simulink model "VTOL"  (R2015b)
settings: Solver=FixedStepAuto  StartTime=0.0  StopTime=30  FixedStep=sampleTime  RelTol=1e-3
InitFcn:
  | sampleTime = 0.01;
  | Ktd = 0.0526/1000;
  | Kdd = 0.0526/1000;
  | Lb = [0.27 0.27 0.27 0.27];
  | LbAssimetrico  = [0.27 0.27 0.18 0.36];
  | LbTeste  = [0.27 0.27 0.18 0.36];
  | Ixx = 0.0754483;
  | Iyy = 0.13642;
  | Izz = 0.2043333;
  | 
  | IXYZ = [Ixx 0 0; 0 Iyy 0; 0 0 Izz];
  | 
  | areaLateral = [0.0114398 0 0; 0 0.09533687 0; 0 0 0.33];
  | 
  | areaAsa = 0.243;
  | areaProfundor = 0.051;
  | densidadeAr = 1.2;
  | cdArrastoParasita = 1.5;
  | clAviao = 0.825;
  | cdAviao = 0.0743;
  | g = 9.8;
  | massa = 3;
  | velCruzeiro = 15;
  | 
  | inicioTransicao = 5;
  | 
  | global kroll
  | global kpitch
  | global kyaw
  | 
  | global kx
  | global ky
  | global kz
undefined symbols (not defined in the file or in its folder): DiscIntNeverNeededParam, kpitch, kroll, kx, ky, kyaw, kz
libraries: simulink x6, aerolibwind2 x1
settings Model: Creator=Avell-G1711  LastModifiedBy=Avell-G1711

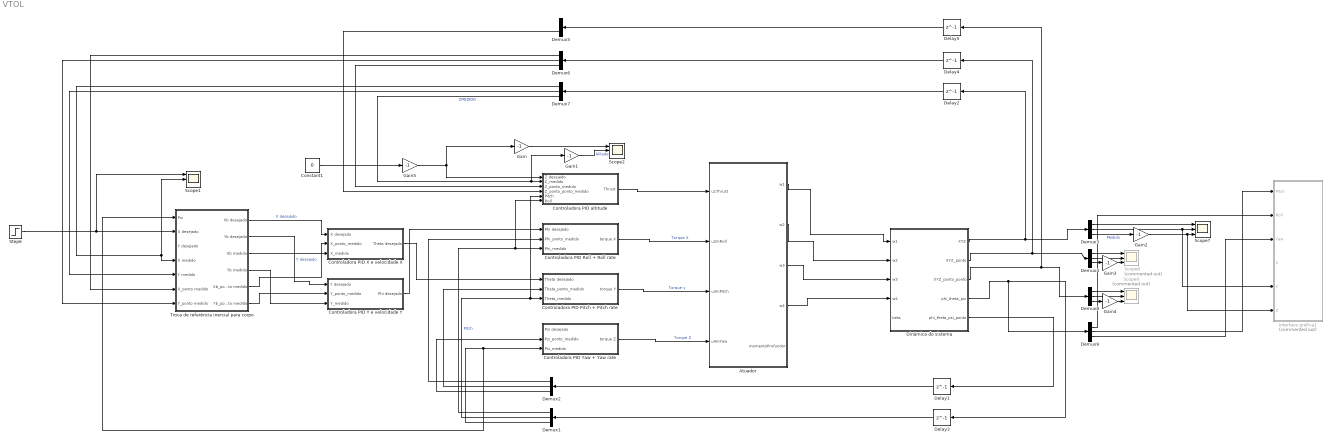
== system VTOL ==
  Atuador : Subsystem
  Constant1 : Constant  Value=0
  Controladora PID Pitch + Pitch rate : Subsystem
  Controladora PID Roll + Roll rate : Subsystem
  Controladora PID X e velocidade X : Subsystem
  Controladora PID Y e velocidade Y : Subsystem
  Controladora PID Yaw + Yaw rate : Subsystem
  Controladora PID altitude : Subsystem
  Delay{1..5} (5 alike) : Delay  DelayLength=1  InitialCondition=[0 0 0]
  Demux{1..9} (9 alike) : Demux  Outputs=3
  Dinâmica do sistema : Subsystem
  Gain{,1..5} (6 alike) : Gain  Gain=-1
  Interface gráfica1 : Subsystem  Commented=on  AncestorBlock=vampLib/Interface gráfica
  Scope1 : Scope  NumInputPorts=3
  Scope2 : Scope  NumInputPorts=3
  Scope7 : Scope  NumInputPorts=3
  Scope8 : Scope  Commented=on  NumInputPorts=3
  Scope9 : Scope  Commented=on  NumInputPorts=3
  Step6 : Step  Time=0  After=20  SampleTime=0
  Troca de referência inercial para corpo : Subsystem
  wires:
  Demux3/1 -> Scope7/1
  Demux3/3 -> Gain2/1  "Medido"
  Demux4/1 -> Scope8/1
  Demux4/2 -> Scope8/2
  Demux4/3 -> Gain3/1
  Dinâmica do sistema/2(XYZ_ponto) -> Delay4/1, Demux4/1
  Dinâmica do sistema/4(phi_theta_psi) -> Demux9/1, Delay3/1
  Dinâmica do sistema/5(phi_theta_psi_ponto) -> Delay1/1
  Delay1/1 -> Demux2/1
  Demux2/1 -> Controladora PID Roll + Roll rate/2(Phi_ponto_medido)
  Demux2/2 -> Controladora PID Pitch + Pitch rate/2(Theta_ponto_medido)
  Demux2/3 -> Controladora PID Yaw + Yaw rate/2(Psi_ponto_medido)
  Demux1/1 -> Controladora PID altitude/6(Roll), Controladora PID Roll + Roll rate/3(Phi_medido)
  Demux1/2 -> Controladora PID altitude/5(Pitch), Controladora PID Pitch + Pitch rate/3(Theta_medido)  "Pitch"
  Atuador/3(w3) -> Dinâmica do sistema/3(w3)
  Atuador/1(w1) -> Dinâmica do sistema/1(w1)
  Atuador/2(w2) -> Dinâmica do sistema/2(w2)
  Atuador/4(w4) -> Dinâmica do sistema/4(w4)
  Controladora PID Roll + Roll rate/1(torque X) -> Atuador/2(u2mRoll)  "Torque X"
  Controladora PID Pitch + Pitch rate/1(torque Y) -> Atuador/3(u3mPitch)  "Torque y"
  Controladora PID Yaw + Yaw rate/1(torque Z) -> Atuador/4(u4mYaw)  "Torque Z"
  Demux7/3 -> Controladora PID altitude/2(Z_medido), Gain1/1  "ZMEDIDO"
  Dinâmica do sistema/1(XYZ) -> Delay2/1, Demux3/1
  Delay5/1 -> Demux5/1
  Delay4/1 -> Demux6/1
  Delay2/1 -> Demux7/1
  Demux5/3 -> Controladora PID altitude/4(Z_ponto_ponto_medido)
  Demux6/3 -> Controladora PID altitude/3(Z_ponto_medido)
  Troca de referência inercial para corpo/1(Xb desejado) -> Controladora PID X e velocidade X/1(X desejado)  "X desejado"
  Troca de referência inercial para corpo/2(Yb desejado) -> Controladora PID Y e velocidade Y/1(Y desejado)  "Y desejado"
  Demux7/1 -> Troca de referência inercial para corpo/4(X medido), Scope1/2
  Demux6/1 -> Troca de referência inercial para corpo/6(X_ponto medido)
  Demux6/2 -> Troca de referência inercial para corpo/7(Y_ponto medido)
  Demux8/1 -> Scope9/1
  Demux8/2 -> Scope9/2
  Demux8/3 -> Gain4/1
  Dinâmica do sistema/3(XYZ_ponto_ponto) -> Demux8/1, Delay5/1
  Gain/1 -> Scope2/1
  Gain1/1 -> Scope2/2  "Alitude"
  Gain2/1 -> Interface gráfica1/6(Z), Scope7/3
  Gain3/1 -> Scope8/3
  Gain4/1 -> Scope9/3
  Troca de referência inercial para corpo/3(Xb medido) -> Controladora PID X e velocidade X/3(X_medido)
  Troca de referência inercial para corpo/4(Yb medido) -> Controladora PID Y e velocidade Y/3(Y_medido)
  Troca de referência inercial para corpo/5(Xb_ponto medido) -> Controladora PID X e velocidade X/2(X_ponto_medido)
  Troca de referência inercial para corpo/6(Yb_ponto medido) -> Controladora PID Y e velocidade Y/2(Y_ponto_medido)
  Demux9/1 -> Interface gráfica1/2(Roll)
  Demux9/3 -> Interface gráfica1/3(Yaw)
  Controladora PID altitude/1(Thrust) -> Atuador/1(u1Thrust)
  Delay3/1 -> Demux1/1
  Demux1/3 -> Troca de referência inercial para corpo/1(Psi), Controladora PID Yaw + Yaw rate/3(Psi_medido)
  Gain5/1 -> Controladora PID altitude/1(Z desejado), Gain/1
  Demux7/2 -> Troca de referência inercial para corpo/5(Y medido)
  Controladora PID X e velocidade X/1(Theta desejado) -> Controladora PID Pitch + Pitch rate/1(Theta desejado)
  Controladora PID Y e velocidade Y/1(Phi desejado) -> Controladora PID Roll + Roll rate/1(Phi desejado)
  Constant1/1 -> Gain5/1
  Demux3/2 -> Interface gráfica1/5(Y), Scope7/2
  Demux9/2 -> Interface gráfica1/1(Pitch)
  Step6/1 -> Troca de referência inercial para corpo/2(X desejado), Scope1/1

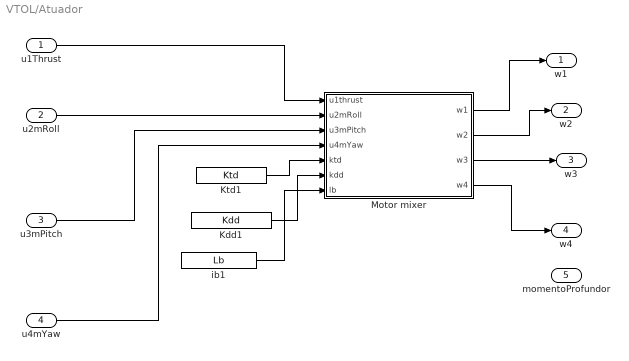
== system VTOL/Atuador ==
  u1Thrust : Inport
  u2mRoll : Inport  Port=2
  u3mPitch : Inport  Port=3
  u4mYaw : Inport  Port=4
  Kdd1 : Constant  Value=Kdd
  Ktd1 : Constant  Value=Ktd
  Motor mixer : MATLAB Function  TreatAsAtomicUnit=on
  ib1 : Constant  Value=Lb
  w1 : Outport
  w2 : Outport  Port=2
  w3 : Outport  Port=3
  w4 : Outport  Port=4
  momentoProfundor : Outport  Port=5
  wires:
  u3mPitch/1 -> Motor mixer/3(u3mPitch)
  ib1/1 -> Motor mixer/7(lb)
  Motor mixer/2(w2) -> w2/1
  Motor mixer/1(w1) -> w1/1
  u1Thrust/1 -> Motor mixer/1(u1thrust)
  Motor mixer/3(w3) -> w3/1
  Motor mixer/4(w4) -> w4/1
  u4mYaw/1 -> Motor mixer/4(u4mYaw)
  u2mRoll/1 -> Motor mixer/2(u2mRoll)
  Ktd1/1 -> Motor mixer/5(ktd)
  Kdd1/1 -> Motor mixer/6(kdd)
  ? -> momentoProfundor/1

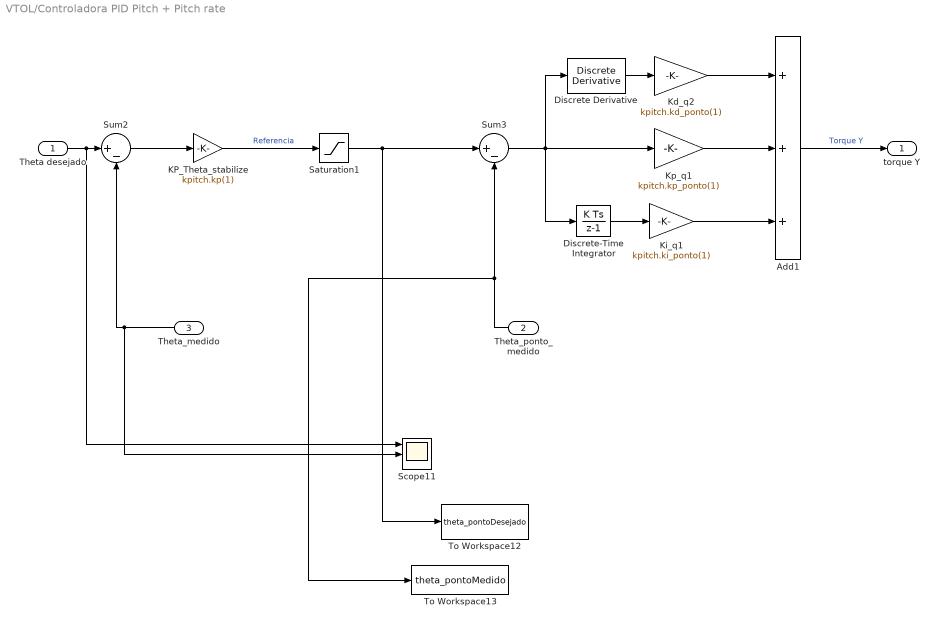
== system VTOL/Controladora PID Pitch + Pitch rate ==
  Theta desejado : Inport
  Theta_ponto_medido : Inport  Port=2
  Theta_medido : Inport  Port=3
  Add1 : Sum  Inputs=+++
  Discrete Derivative : simulink/Discrete/Discrete Derivative  gainval=1.0  ICPrevScaledInput=0.0  InputProcessing=Inherited  OutMin=[]  OutMax=[]  OutDataType=fixdt(1, 16)  OutScaling=2^-10  DoSatur=off
  Discrete-Time Integrator : DiscreteIntegrator  InitialConditionSetting=State (most efficient)  SampleTime=-1  ICPrevOutput=DiscIntNeverNeededParam  ICPrevScaledInput=DiscIntNeverNeededParam
  KP_Theta_stabilize : Gain  Gain=kpitch.kp(1)
  Kd_q2 : Gain  Gain=kpitch.kd_ponto(1)
  Ki_q1 : Gain  Gain=kpitch.ki_ponto(1)
  Kp_q1 : Gain  Gain=kpitch.kp_ponto(1)
  Saturation1 : Saturate  UpperLimit=2*pi  LowerLimit=-2*pi
  Scope11 : Scope  NumInputPorts=3
  Sum2 : Sum  Inputs=|+-
  Sum3 : Sum  Inputs=|+-
  To Workspace12 : ToWorkspace  VariableName=theta_pontoDesejado  SaveFormat=Timeseries  SampleTime=-1
  To Workspace13 : ToWorkspace  VariableName=theta_pontoMedido  SaveFormat=Timeseries  SampleTime=-1
  torque Y : Outport
  wires:
  Theta_ponto_medido/1 -> To Workspace13/1, Sum3/2
  Discrete-Time Integrator/1 -> Ki_q1/1
  Theta_medido/1 -> Scope11/2, Sum2/2
  Kd_q2/1 -> Add1/1
  Sum2/1 -> KP_Theta_stabilize/1
  Ki_q1/1 -> Add1/3
  Discrete Derivative/1 -> Kd_q2/1
  Sum3/1 -> Discrete Derivative/1, Discrete-Time Integrator/1, Kp_q1/1
  Kp_q1/1 -> Add1/2
  Theta desejado/1 -> Scope11/1, Sum2/1
  KP_Theta_stabilize/1 -> Saturation1/1  "Referencia"
  Add1/1 -> torque Y/1  "Torque Y"
  Saturation1/1 -> To Workspace12/1, Sum3/1

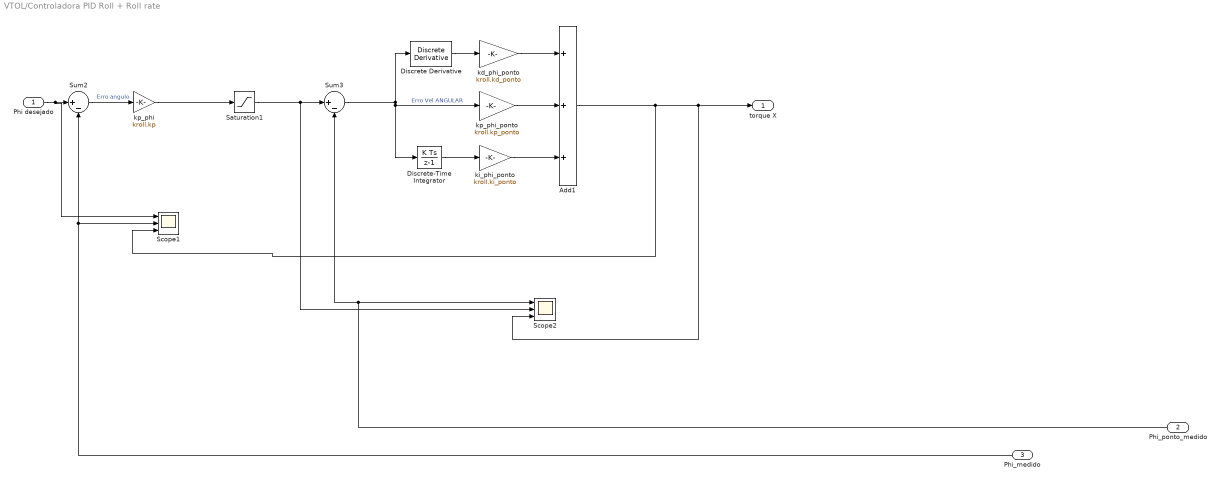
== system VTOL/Controladora PID Roll + Roll rate ==
  Phi desejado : Inport
  Phi_ponto_medido : Inport  Port=2
  Phi_medido : Inport  Port=3
  Add1 : Sum  Inputs=+++
  Discrete Derivative : simulink/Discrete/Discrete Derivative  gainval=1.0  ICPrevScaledInput=0.0  InputProcessing=Inherited  OutMin=[]  OutMax=[]  OutDataType=fixdt(1, 16)  OutScaling=2^-10  DoSatur=off
  Discrete-Time Integrator : DiscreteIntegrator  InitialConditionSetting=State (most efficient)  SampleTime=-1  ICPrevOutput=DiscIntNeverNeededParam  ICPrevScaledInput=DiscIntNeverNeededParam
  Saturation1 : Saturate  UpperLimit=2*pi  LowerLimit=-2*pi
  Scope1 : Scope  NumInputPorts=3
  Scope2 : Scope  NumInputPorts=3
  Sum2 : Sum  Inputs=|+-
  Sum3 : Sum  Inputs=|+-
  kd_phi_ponto : Gain  Gain=kroll.kd_ponto
  ki_phi_ponto : Gain  Gain=kroll.ki_ponto
  kp_phi : Gain  Gain=kroll.kp
  kp_phi_ponto : Gain  Gain=kroll.kp_ponto
  torque X : Outport
  wires:
  Phi_ponto_medido/1 -> Sum3/2, Scope2/1
  Discrete-Time Integrator/1 -> ki_phi_ponto/1
  Add1/1 -> Scope1/3, Scope2/3, torque X/1
  kd_phi_ponto/1 -> Add1/1
  Sum2/1 -> kp_phi/1  "Erro angulo"
  ki_phi_ponto/1 -> Add1/3
  Discrete Derivative/1 -> kd_phi_ponto/1
  kp_phi_ponto/1 -> Add1/2
  Phi desejado/1 -> Scope1/1, Sum2/1
  Sum3/1 -> Discrete-Time Integrator/1, kp_phi_ponto/1, Discrete Derivative/1  "Erro Vel ANGULAR"
  Phi_medido/1 -> Scope1/2, Sum2/2
  kp_phi/1 -> Saturation1/1
  Saturation1/1 -> Scope2/2, Sum3/1

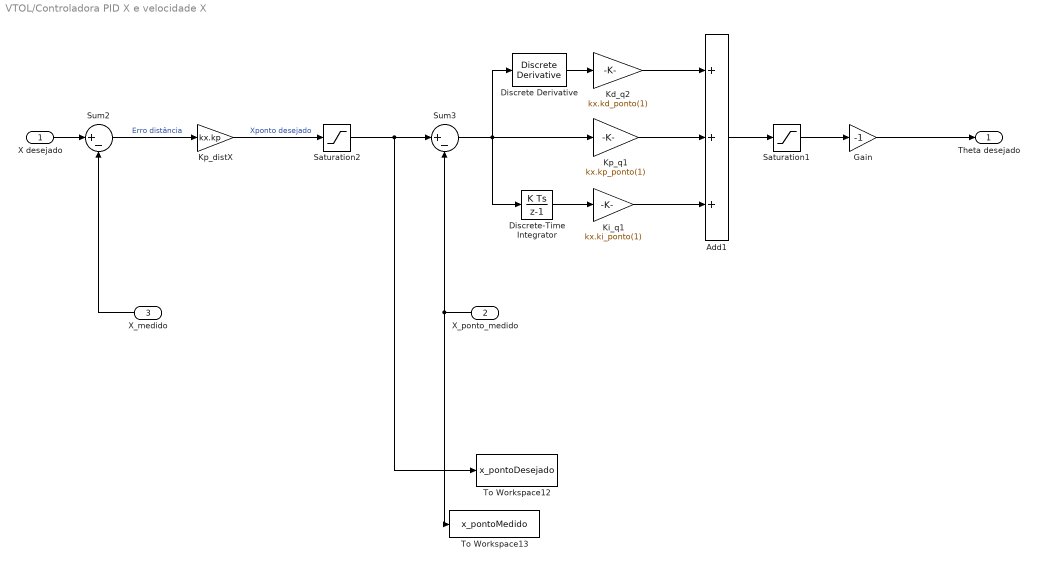
== system VTOL/Controladora PID X e velocidade X ==
  X desejado : Inport
  X_ponto_medido : Inport  Port=2
  X_medido : Inport  Port=3
  Add1 : Sum  Inputs=+++
  Discrete Derivative : simulink/Discrete/Discrete Derivative  gainval=1.0  ICPrevScaledInput=0.0  InputProcessing=Inherited  OutMin=[]  OutMax=[]  OutDataType=fixdt(1, 16)  OutScaling=2^-10  DoSatur=off
  Discrete-Time Integrator : DiscreteIntegrator  InitialConditionSetting=State (most efficient)  SampleTime=-1  ICPrevOutput=DiscIntNeverNeededParam  ICPrevScaledInput=DiscIntNeverNeededParam
  Gain : Gain  Gain=-1
  Kd_q2 : Gain  Gain=kx.kd_ponto(1)
  Ki_q1 : Gain  Gain=kx.ki_ponto(1)
  Kp_distX : Gain  Gain=kx.kp
  Kp_q1 : Gain  Gain=kx.kp_ponto(1)
  Saturation1 : Saturate  UpperLimit=0.7  LowerLimit=-0.7
  Saturation2 : Saturate  UpperLimit=4  LowerLimit=-4
  Sum2 : Sum  Inputs=|+-
  Sum3 : Sum  Inputs=|+-
  To Workspace12 : ToWorkspace  VariableName=x_pontoDesejado  SaveFormat=Timeseries  SampleTime=-1
  To Workspace13 : ToWorkspace  VariableName=x_pontoMedido  SaveFormat=Timeseries  SampleTime=-1
  Theta desejado : Outport
  wires:
  X_ponto_medido/1 -> Sum3/2, To Workspace13/1
  Discrete-Time Integrator/1 -> Ki_q1/1
  Add1/1 -> Saturation1/1
  Kd_q2/1 -> Add1/1
  Sum2/1 -> Kp_distX/1  "Erro distância"
  Ki_q1/1 -> Add1/3
  Discrete Derivative/1 -> Kd_q2/1
  Kp_q1/1 -> Add1/2
  X desejado/1 -> Sum2/1
  Kp_distX/1 -> Saturation2/1  "Xponto desejado"
  Sum3/1 -> Discrete Derivative/1, Discrete-Time Integrator/1, Kp_q1/1
  X_medido/1 -> Sum2/2
  Saturation1/1 -> Gain/1
  Saturation2/1 -> To Workspace12/1, Sum3/1
  Gain/1 -> Theta desejado/1

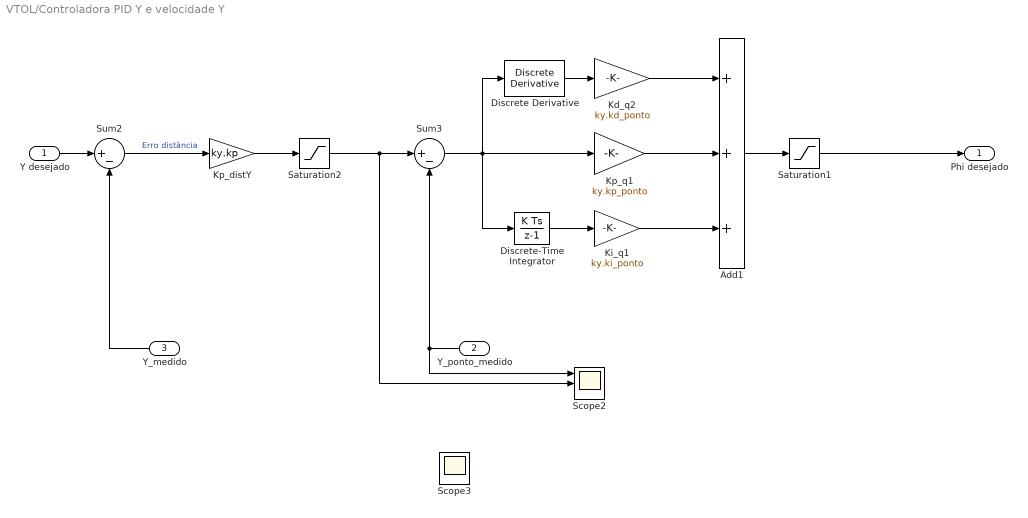
== system VTOL/Controladora PID Y e velocidade Y ==
  Y desejado : Inport
  Y_ponto_medido : Inport  Port=2
  Y_medido : Inport  Port=3
  Add1 : Sum  Inputs=+++
  Discrete Derivative : simulink/Discrete/Discrete Derivative  gainval=1.0  ICPrevScaledInput=0.0  InputProcessing=Inherited  OutMin=[]  OutMax=[]  OutDataType=fixdt(1, 16)  OutScaling=2^-10  DoSatur=off
  Discrete-Time Integrator : DiscreteIntegrator  InitialConditionSetting=State (most efficient)  SampleTime=-1  ICPrevOutput=DiscIntNeverNeededParam  ICPrevScaledInput=DiscIntNeverNeededParam
  Kd_q2 : Gain  Gain=ky.kd_ponto
  Ki_q1 : Gain  Gain=ky.ki_ponto
  Kp_distY : Gain  Gain=ky.kp
  Kp_q1 : Gain  Gain=ky.kp_ponto
  Saturation1 : Saturate  UpperLimit=0.7  LowerLimit=-0.7
  Saturation2 : Saturate  UpperLimit=4  LowerLimit=-4
  Scope2 : Scope  NumInputPorts=3
  Scope3 : Scope  NumInputPorts=3
  Sum2 : Sum  Inputs=|+-
  Sum3 : Sum  Inputs=|+-
  Phi desejado : Outport
  wires:
  Y_ponto_medido/1 -> Sum3/2, Scope2/1
  Discrete-Time Integrator/1 -> Ki_q1/1
  Add1/1 -> Saturation1/1
  Kd_q2/1 -> Add1/1
  Sum2/1 -> Kp_distY/1  "Erro distância"
  Ki_q1/1 -> Add1/3
  Discrete Derivative/1 -> Kd_q2/1
  Kp_q1/1 -> Add1/2
  Y desejado/1 -> Sum2/1
  Kp_distY/1 -> Saturation2/1
  Sum3/1 -> Discrete Derivative/1, Discrete-Time Integrator/1, Kp_q1/1
  Y_medido/1 -> Sum2/2
  Saturation2/1 -> Scope2/2, Sum3/1
  Saturation1/1 -> Phi desejado/1

== system VTOL/Controladora PID Yaw + Yaw rate ==
  Psi desejado : Inport
  Psi_ponto_medido : Inport  Port=2
  Psi_medido : Inport  Port=3
  Add1 : Sum  Inputs=+++
  Discrete Derivative : simulink/Discrete/Discrete Derivative  gainval=1.0  ICPrevScaledInput=0.0  InputProcessing=Inherited  OutMin=[]  OutMax=[]  OutDataType=fixdt(1, 16)  OutScaling=2^-10  DoSatur=off
  Discrete-Time Integrator : DiscreteIntegrator  InitialConditionSetting=State (most efficient)  SampleTime=-1  ICPrevOutput=DiscIntNeverNeededParam  ICPrevScaledInput=DiscIntNeverNeededParam
  KP_phi_stabilize1 : Gain  Gain=kyaw.kp
  Kd_q2 : Gain  Gain=kyaw.kd_ponto
  Ki_q1 : Gain  Gain=kyaw.ki_ponto
  Kp_q1 : Gain  Gain=kyaw.kp_ponto
  Sum2 : Sum  Inputs=|+-
  Sum3 : Sum  Inputs=|+-
  torque Z : Outport
  wires:
  Psi_ponto_medido/1 -> Sum3/2
  Discrete-Time Integrator/1 -> Ki_q1/1
  Psi_medido/1 -> Sum2/2
  Kd_q2/1 -> Add1/1
  Sum2/1 -> KP_phi_stabilize1/1
  Ki_q1/1 -> Add1/3
  Discrete Derivative/1 -> Kd_q2/1
  Sum3/1 -> Discrete Derivative/1, Discrete-Time Integrator/1, Kp_q1/1
  Kp_q1/1 -> Add1/2
  Psi desejado/1 -> Sum2/1
  KP_phi_stabilize1/1 -> Sum3/1  "Referencia"
  Add1/1 -> torque Z/1  "Torque Z"

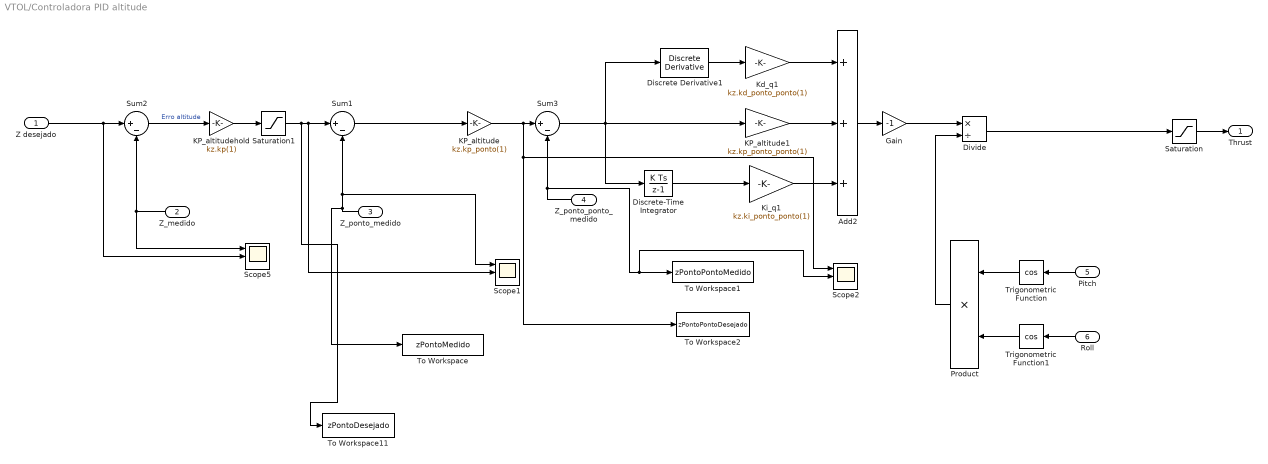
== system VTOL/Controladora PID altitude ==
  Z desejado : Inport
  Z_medido : Inport  Port=2
  Z_ponto_medido : Inport  Port=3
  Z_ponto_ponto_medido : Inport  Port=4
  Pitch : Inport  Port=5
  Roll : Inport  Port=6
  Add2 : Sum  Inputs=+++
  Discrete Derivative1 : simulink/Discrete/Discrete Derivative  gainval=1.0  ICPrevScaledInput=0.0  InputProcessing=Inherited  OutMin=[]  OutMax=[]  OutDataType=fixdt(1, 16)  OutScaling=2^-10  DoSatur=off
  Discrete-Time Integrator : DiscreteIntegrator  InitialConditionSetting=State (most efficient)  SampleTime=-1  ICPrevOutput=DiscIntNeverNeededParam  ICPrevScaledInput=DiscIntNeverNeededParam
  Divide : Product  Inputs=*/
  Gain : Gain  Gain=-1
  KP_altitude : Gain  Gain=kz.kp_ponto(1)
  KP_altitude1 : Gain  Gain=kz.kp_ponto_ponto(1)
  KP_altitudehold : Gain  Gain=kz.kp(1)
  Kd_q1 : Gain  Gain=kz.kd_ponto_ponto(1)
  Ki_q1 : Gain  Gain=kz.ki_ponto_ponto(1)
  Product : Product
  Saturation : Saturate  UpperLimit=53  LowerLimit=0
  Saturation1 : Saturate  UpperLimit=2  LowerLimit=-2
  Scope1 : Scope  NumInputPorts=3
  Scope2 : Scope  NumInputPorts=3
  Scope5 : Scope  NumInputPorts=3
  Sum1 : Sum  Inputs=|+-
  Sum2 : Sum  Inputs=|+-
  Sum3 : Sum  Inputs=|+-
  To Workspace : ToWorkspace  VariableName=zPontoMedido  SaveFormat=Timeseries  SampleTime=-1
  To Workspace1 : ToWorkspace  VariableName=zPontoPontoMedido  SaveFormat=Timeseries  SampleTime=-1
  To Workspace11 : ToWorkspace  VariableName=zPontoDesejado  SaveFormat=Timeseries  SampleTime=-1
  To Workspace2 : ToWorkspace  VariableName=zPontoPontoDesejado  SaveFormat=Timeseries  SampleTime=-1
  Trigonometric Function : Trigonometry  Operator=cos
  Trigonometric Function1 : Trigonometry  Operator=cos
  Thrust : Outport
  wires:
  Sum2/1 -> KP_altitudehold/1  "Erro altitude"
  Z desejado/1 -> Scope5/2, Sum2/1
  Z_medido/1 -> Sum2/2, Scope5/1
  Z_ponto_medido/1 -> To Workspace/1, Scope1/1, Sum1/2
  KP_altitudehold/1 -> Saturation1/1
  Sum1/1 -> KP_altitude/1
  KP_altitude/1 -> Scope2/1, To Workspace2/1, Sum3/1
  Z_ponto_ponto_medido/1 -> Scope2/2, To Workspace1/1, Sum3/2
  KP_altitude1/1 -> Add2/2
  Discrete Derivative1/1 -> Kd_q1/1
  Kd_q1/1 -> Add2/1
  Discrete-Time Integrator/1 -> Ki_q1/1
  Ki_q1/1 -> Add2/3
  Sum3/1 -> Discrete-Time Integrator/1, KP_altitude1/1, Discrete Derivative1/1
  Pitch/1 -> Trigonometric Function/1
  Roll/1 -> Trigonometric Function1/1
  Product/1 -> Divide/2
  Add2/1 -> Gain/1
  Trigonometric Function/1 -> Product/1
  Trigonometric Function1/1 -> Product/2
  Gain/1 -> Divide/1
  Saturation/1 -> Thrust/1
  Divide/1 -> Saturation/1
  Saturation1/1 -> To Workspace11/1, Scope1/2, Sum1/1

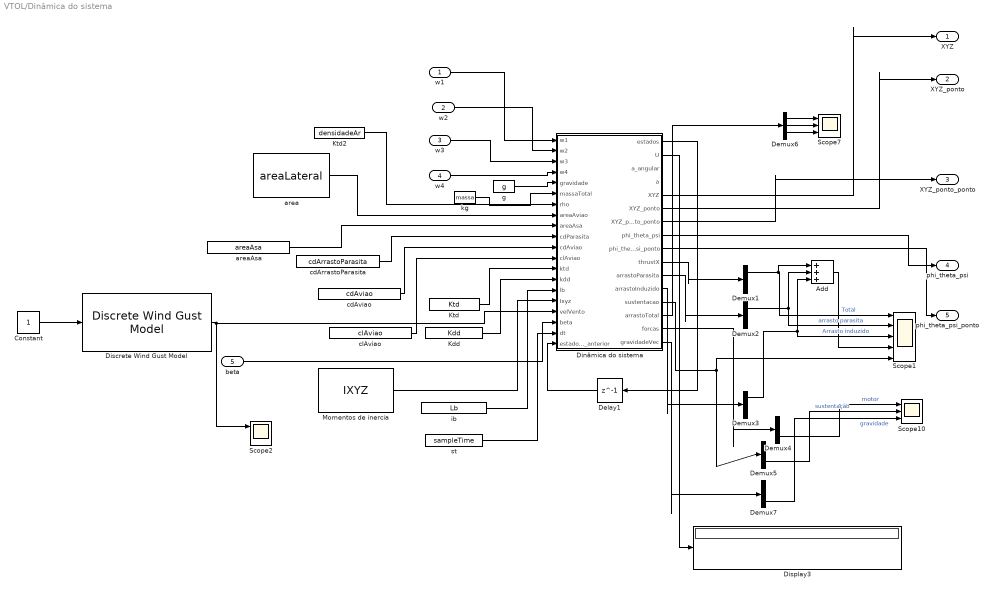
== system VTOL/Dinâmica do sistema ==
  w1 : Inport
  w2 : Inport  Port=2
  w3 : Inport  Port=3
  w4 : Inport  Port=4
  beta : Inport  Port=5
  Add : Sum  Inputs=+++
  Constant : Constant
  Delay1 : Delay  DelayLength=1  InitialCondition=[0 0 0 0;0 0 0 0;0 0 0 0]
  Demux{1..7} (7 alike) : Demux  Outputs=3
  Dinâmica do sistema : MATLAB Function  TreatAsAtomicUnit=on
  Discrete Wind Gust Model : aerolibwind2/Discrete Wind Gust Model  units=Metric (MKS)  Gx=on  Gy=on  Gz=on  t_0=10  d_m=[10 10 10]  v_m=[0 0 0]
  Display3 : Display
  Kdd : Constant  Value=Kdd
  Ktd : Constant  Value=Ktd
  Ktd2 : Constant  Value=densidadeAr
  Momentos de inercia : Constant  Value=IXYZ
  Scope1 : Scope  NumInputPorts=5
  Scope10 : Scope  NumInputPorts=3
  Scope2 : Scope  NumInputPorts=3
  Scope7 : Scope  NumInputPorts=3
  "area " : Constant  Value=areaLateral
  areaAsa : Constant  Value=areaAsa
  cdArrastoParasita : Constant  Value=cdArrastoParasita
  cdAviao : Constant  Value=cdAviao
  clAviao : Constant  Value=clAviao
  g : Constant  Value=g  SampleTime=sampleTime
  ib : Constant  Value=Lb
  kg : Constant  Value=massa  SampleTime=sampleTime
  st : Constant  Value=sampleTime
  XYZ : Outport
  XYZ_ponto : Outport  Port=2
  XYZ_ponto_ponto : Outport  Port=3
  phi_theta_psi : Outport  Port=4
  phi_theta_psi_ponto : Outport  Port=5
  wires:
  Dinâmica do sistema/1(estados) -> Delay1/1
  Delay1/1 -> Dinâmica do sistema/20(estados_anterior)
  ib/1 -> Dinâmica do sistema/15(lb)
  Momentos de inercia/1 -> Dinâmica do sistema/16(Ixyz)
  st/1 -> Dinâmica do sistema/19(dt)
  Kdd/1 -> Dinâmica do sistema/14(kdd)
  kg/1 -> Dinâmica do sistema/6(massaTotal)
  g/1 -> Dinâmica do sistema/5(gravidade)
  Ktd/1 -> Dinâmica do sistema/13(ktd)
  Dinâmica do sistema/5(XYZ) -> XYZ/1
  w3/1 -> Dinâmica do sistema/3(w3)
  w4/1 -> Dinâmica do sistema/4(w4)
  Dinâmica do sistema/6(XYZ_ponto) -> XYZ_ponto/1
  w2/1 -> Dinâmica do sistema/2(w2)
  Dinâmica do sistema/9(phi_theta_psi_ponto) -> phi_theta_psi_ponto/1
  Dinâmica do sistema/8(phi_theta_psi) -> phi_theta_psi/1
  w1/1 -> Dinâmica do sistema/1(w1)
  Dinâmica do sistema/2(U) -> Display3/1
  "area "/1 -> Dinâmica do sistema/8(areaAviao)
  cdArrastoParasita/1 -> Dinâmica do sistema/10(cdParasita)
  Ktd2/1 -> Dinâmica do sistema/7(rho)
  cdAviao/1 -> Dinâmica do sistema/11(cdAviao)
  clAviao/1 -> Dinâmica do sistema/12(clAviao)
  areaAsa/1 -> Dinâmica do sistema/9(areaAsa)
  Demux6/1 -> Scope7/1
  Demux6/2 -> Scope7/2
  Demux6/3 -> Scope7/3
  Dinâmica do sistema/14(arrastoTotal) -> Demux6/1
  beta/1 -> Dinâmica do sistema/18(beta)
  Dinâmica do sistema/10(thrustX) -> Demux1/1
  Dinâmica do sistema/11(arrastoParasita) -> Demux2/1
  Dinâmica do sistema/12(arrastoInduzido) -> Demux3/1
  Demux1/1 -> Add/1, Scope1/1
  Demux2/1 -> Add/2, Scope1/2  "arrasto parasita"
  Demux3/1 -> Add/3, Scope1/3  "Arrasto induzido"
  Add/1 -> Scope1/4  "Total"
  Dinâmica do sistema/13(sustentacao) -> Demux5/1, Scope1/5
  Dinâmica do sistema/15(forcas) -> Demux4/1
  Demux4/3 -> Scope10/1  "motor"
  Demux5/3 -> Scope10/2  "sustentação"
  Dinâmica do sistema/16(gravidadeVec) -> Demux7/1
  Demux7/3 -> Scope10/3  "gravidade"
  Dinâmica do sistema/7(XYZ_ponto_ponto) -> XYZ_ponto_ponto/1
  Discrete Wind Gust Model/1 -> Scope2/1, Dinâmica do sistema/17(velVento)
  Constant/1 -> Discrete Wind Gust Model/1

== system VTOL/Interface gráfica1 ==
  Pitch : Inport
  Roll : Inport  Port=2
  Yaw : Inport  Port=3
  X : Inport  Port=4
  Y : Inport  Port=5
  Z : Inport  Port=6
  Desenho do drone : MATLAB Function  TreatAsAtomicUnit=on
  Display : Display  Commented=on
  Display1 : Display  Commented=on
  Rotacao : MATLAB Function  TreatAsAtomicUnit=on
  Vector Concatenate : Concatenate  NumInputs=3
  Vector Concatenate1 : Concatenate  NumInputs=3
  desenhaVetores : MATLAB Function  TreatAsAtomicUnit=on
  wires:
  Roll/1 -> Vector Concatenate/2
  Z/1 -> Vector Concatenate1/3
  Y/1 -> Vector Concatenate1/2
  X/1 -> Vector Concatenate1/1
  Vector Concatenate/1 -> Rotacao/2(PitchRollYaw), Display/1
  Pitch/1 -> Vector Concatenate/1
  Yaw/1 -> Vector Concatenate/3
  Rotacao/1(vetorNoEixoInercial) -> desenhaVetores/2(vetorNoEixoInercial)
  Vector Concatenate1/1 -> Display1/1, Rotacao/3(XYZ)
  Desenho do drone/1(desenhoDrone) -> Rotacao/1(vetorNoEixoDoCorpo), desenhaVetores/1(vetorNoEixoDoCorpo)

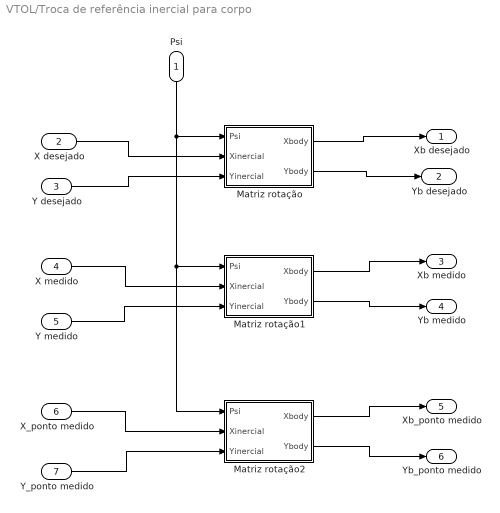
== system VTOL/Troca de referência inercial para corpo ==
  Psi : Inport
  X desejado : Inport  Port=2
  Y desejado : Inport  Port=3
  X medido : Inport  Port=4
  Y medido : Inport  Port=5
  X_ponto medido : Inport  Port=6
  Y_ponto medido : Inport  Port=7
  Matriz rotação : Subsystem
  Matriz rotação1 : Subsystem
  Matriz rotação2 : Subsystem
  Xb desejado : Outport
  Yb desejado : Outport  Port=2
  Xb medido : Outport  Port=3
  Yb medido : Outport  Port=4
  Xb_ponto medido : Outport  Port=5
  Yb_ponto medido : Outport  Port=6
  wires:
  Psi/1 -> Matriz rotação2/1(Psi), Matriz rotação1/1(Psi), Matriz rotação/1(Psi)
  X desejado/1 -> Matriz rotação/2(Xinercial)
  Y desejado/1 -> Matriz rotação/3(Yinercial)
  X medido/1 -> Matriz rotação1/2(Xinercial)
  Y medido/1 -> Matriz rotação1/3(Yinercial)
  X_ponto medido/1 -> Matriz rotação2/2(Xinercial)
  Y_ponto medido/1 -> Matriz rotação2/3(Yinercial)
  Matriz rotação/1(Xbody) -> Xb desejado/1
  Matriz rotação/2(Ybody) -> Yb desejado/1
  Matriz rotação1/1(Xbody) -> Xb medido/1
  Matriz rotação1/2(Ybody) -> Yb medido/1
  Matriz rotação2/1(Xbody) -> Xb_ponto medido/1
  Matriz rotação2/2(Ybody) -> Yb_ponto medido/1

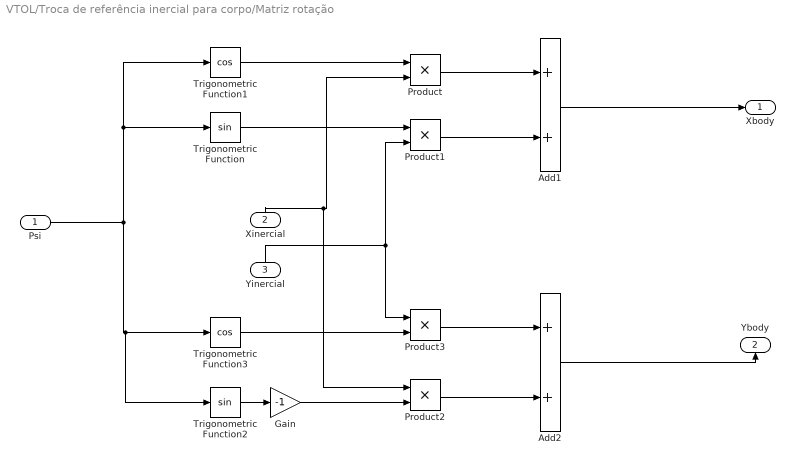
== system VTOL/Troca de referência inercial para corpo/Matriz rotação ==
  Psi : Inport
  Xinercial : Inport  Port=2
  Yinercial : Inport  Port=3
  Add1 : Sum
  Add2 : Sum
  Gain : Gain  Gain=-1
  Product{,1..3} (4 alike) : Product
  Trigonometric Function : Trigonometry
  Trigonometric Function1 : Trigonometry  Operator=cos
  Trigonometric Function2 : Trigonometry
  Trigonometric Function3 : Trigonometry  Operator=cos
  Xbody : Outport
  Ybody : Outport  Port=2
  wires:
  Add1/1 -> Xbody/1
  Product/1 -> Add1/1
  Add2/1 -> Ybody/1
  Yinercial/1 -> Product1/2, Product3/1
  Product3/1 -> Add2/1
  Product2/1 -> Add2/2
  Product1/1 -> Add1/2
  Trigonometric Function3/1 -> Product3/2
  Trigonometric Function1/1 -> Product/1
  Gain/1 -> Product2/2
  Xinercial/1 -> Product2/1, Product/2
  Trigonometric Function2/1 -> Gain/1
  Trigonometric Function/1 -> Product1/1
  Psi/1 -> Trigonometric Function/1, Trigonometric Function1/1, Trigonometric Function2/1, Trigonometric Function3/1

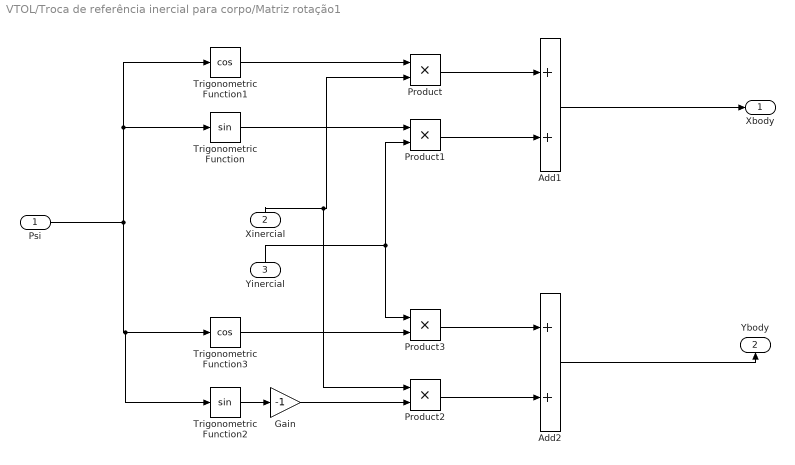
== system VTOL/Troca de referência inercial para corpo/Matriz rotação1 ==
  Psi : Inport
  Xinercial : Inport  Port=2
  Yinercial : Inport  Port=3
  Add1 : Sum
  Add2 : Sum
  Gain : Gain  Gain=-1
  Product{,1..3} (4 alike) : Product
  Trigonometric Function : Trigonometry
  Trigonometric Function1 : Trigonometry  Operator=cos
  Trigonometric Function2 : Trigonometry
  Trigonometric Function3 : Trigonometry  Operator=cos
  Xbody : Outport
  Ybody : Outport  Port=2
  wires:
  Add1/1 -> Xbody/1
  Product/1 -> Add1/1
  Add2/1 -> Ybody/1
  Yinercial/1 -> Product1/2, Product3/1
  Product3/1 -> Add2/1
  Product2/1 -> Add2/2
  Product1/1 -> Add1/2
  Trigonometric Function3/1 -> Product3/2
  Trigonometric Function1/1 -> Product/1
  Gain/1 -> Product2/2
  Xinercial/1 -> Product2/1, Product/2
  Trigonometric Function2/1 -> Gain/1
  Trigonometric Function/1 -> Product1/1
  Psi/1 -> Trigonometric Function/1, Trigonometric Function1/1, Trigonometric Function2/1, Trigonometric Function3/1

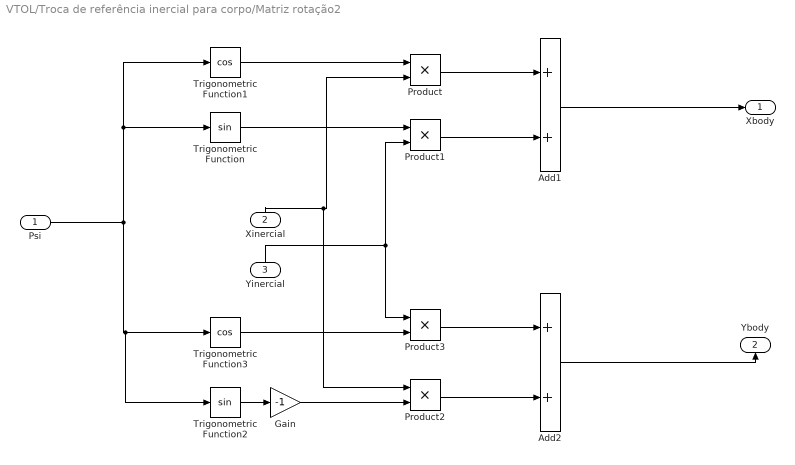
== system VTOL/Troca de referência inercial para corpo/Matriz rotação2 ==
  Psi : Inport
  Xinercial : Inport  Port=2
  Yinercial : Inport  Port=3
  Add1 : Sum
  Add2 : Sum
  Gain : Gain  Gain=-1
  Product{,1..3} (4 alike) : Product
  Trigonometric Function : Trigonometry
  Trigonometric Function1 : Trigonometry  Operator=cos
  Trigonometric Function2 : Trigonometry
  Trigonometric Function3 : Trigonometry  Operator=cos
  Xbody : Outport
  Ybody : Outport  Port=2
  wires:
  Add1/1 -> Xbody/1
  Product/1 -> Add1/1
  Add2/1 -> Ybody/1
  Yinercial/1 -> Product1/2, Product3/1
  Product3/1 -> Add2/1
  Product2/1 -> Add2/2
  Product1/1 -> Add1/2
  Trigonometric Function3/1 -> Product3/2
  Trigonometric Function1/1 -> Product/1
  Gain/1 -> Product2/2
  Xinercial/1 -> Product2/1, Product/2
  Trigonometric Function2/1 -> Gain/1
  Trigonometric Function/1 -> Product1/1
  Psi/1 -> Trigonometric Function/1, Trigonometric Function1/1, Trigonometric Function2/1, Trigonometric Function3/1

== matlab function VTOL/Dinâmica do sistema/Dinâmica do sistema ==
  data: w1 input; w2 input; w3 input; w4 input; estados output; gravidade input; massaTotal input; rho input; areaAviao input; areaAsa input; cdParasita input; cdAviao input; clAviao input; ktd input; kdd input; lb input; Ixyz input; velVento input; beta input; dt input; estados_anterior input; U output; a_angular output; a output; XYZ output; XYZ_ponto output; XYZ_ponto_ponto output; phi_theta_psi output; phi_theta_psi_ponto output; thrustX output; arrastoParasita output; arrastoInduzido output; sustentacao output; arrastoTotal output; forcas output; gravidadeVec output
function [estados, U, a_angular, a, XYZ, XYZ_ponto,XYZ_ponto_ponto, phi_theta_psi, phi_theta_psi_ponto, thrustX, arrastoParasita, arrastoInduzido, sustentacao, arrastoTotal, forcas, gravidadeVec]  = fcn(w1,w2, w3, w4, gravidade, massaTotal,rho,areaAviao, areaAsa, cdParasita, cdAviao, clAviao, ktd, kdd, lb, Ixyz, velVento, beta, dt, estados_anterior)

% Separa entrada nos vetores
XYZ = estados_anterior(:, 1);
XYZ_ponto = estados_anterior(:, 2);
phi_theta_psi = estados_anterior(:, 3);
phi_theta_psi_ponto = estados_anterior(:, 4);

% Relaciona atitudes da aeronave
roll = phi_theta_psi(1);
pitch = phi_theta_psi(2);
yaw = phi_theta_psi(3);
phi = roll;
theta = pitch;
psi = yaw;


% Define Matriz de rotação ZYX 
matrizRotacao =     [cos(theta)*cos(psi) cos(psi)*sin(theta)*sin(phi)-sin(psi)*cos(phi) cos(psi)*sin(theta)*cos(phi)+sin(psi)*sin(phi);
                     sin(psi)*cos(theta) sin(psi)*sin(theta)*sin(phi)+cos(psi)*cos(phi) sin(psi)*sin(theta)*cos(phi)-cos(psi)*sin(phi);
                     -sin(theta) cos(theta)*sin(phi) cos(theta)*cos(phi)];

% Matriz de transformação das velocidades angulares
T = [1 0 -sin(theta);
    0 cos(phi) cos(theta)*sin(phi);
    0 -sin(phi) cos(theta)*cos(phi)];

% Encontra velocidades lineares e angulares no eixo do corpo com base no
% eixo inercial
vel_angular_body = T*phi_theta_psi_ponto;
vel_linear_body = matrizRotacao'*XYZ_ponto;

%Velocidade do vento no referencial do corpo
vel_vento_body = matrizRotacao'*velVento;

% Velocidade do corpo em relação ao vento
vel_aerodinamica_body = vel_linear_body-vel_vento_body;


% Forças e momentos gerados por cada rotação dos motores
w2ParaU = [ ktd      ktd     ktd      ktd;
           -ktd*lb(2)      ktd*lb(1)     ktd*lb(1)     -ktd*lb(2);
            ktd*lb(3)     -ktd*lb(4)     ktd*lb(3)     -ktd*lb(4);
           -kdd     -kdd       kdd      kdd];


% Calcula a força no eixo Z causada pelos motores
U = w2ParaU * [w1^2*cos(beta); w2^2; w3^2*cos(beta); w4^2]; % Componente vertical, motor 1 e 3 estão em tilt com ângulo Beta

% Calcula a força no eixo X causada pelos motores
thrustX = [([ ktd      ktd     ktd      ktd]*[w1^2*sin(beta); 0; w3^2*sin(beta); 0]) ; 0 ; 0];% Componente da força horizontal, com motor tiltado

% Forças presentes no referencial do corpo
thrust = U(1)*[0; 0; 1];
forcas = -thrust;

% Calcula arrasto parasita
arrastoParasita = -sign(vel_aerodinamica_body).*((rho*(vel_aerodinamica_body.^2)'*cdParasita*areaAviao/2)'); % Calcula arrasto parasita

% Calcula arrasto induzido e sustentação se tiver velocidade em X
if(vel_aerodinamica_body(1) > 0)
    arrastoInduzido = [-rho*vel_aerodinamica_body(1)^2*cdAviao*areaAsa/2 ; 0 ; 0]; % Encontra arrasto induzido da asa + profundor (o cd ta ajustado pra usar apenas a área da asa)
    sustentacao = [0 ; 0 ; -rho*vel_aerodinamica_body(1)^2*clAviao*areaAsa/2];
else
     arrastoInduzido = [0;0;0];
     sustentacao = [0;0;0];
end

% Arrasto total
arrastoTotal = arrastoParasita+arrastoInduzido;

% Gravidade
gravidadeVec = (matrizRotacao')*(massaTotal*gravidade*[0; 0; 1]);

% Somatório total de forças
FtotalBody = -thrust + gravidadeVec + arrastoParasita+arrastoInduzido+sustentacao + thrustX; 

% Momentos presentes no body frame axis
% Lembrando que em VTOL se desconsidera o momento do profundor
mXroll = U(2);
mYpitch = U(3);
mZyaw = U(4);
momentos = [mXroll; mYpitch; mZyaw];

% Adiciona efeito giroscópio e efeitos do produto vetorial do modelo de
% Newton-Euler
FtotalBody = FtotalBody - cross(vel_angular_body,(massaTotal*vel_linear_body));
momentos = momentos - cross(vel_angular_body,(Ixyz*vel_angular_body));

% Calcula aceleração em relação ao body frame
a = FtotalBody/massaTotal;

%Calcula aceleração angular em relação ao body frame
a_angular = inv(Ixyz)*(momentos);

% Calcula velocidade angular em relação ao body axis
vel_angular_body = vel_angular_body + a_angular*dt;

% Encontra velocidade angular em relação ao eixo inercial
phi_theta_psi_ponto = inv(T)*vel_angular_body;

% Encontra os ângulos com base na velocidade angular no eixo inercial
phi_theta_psi = phi_theta_psi+ phi_theta_psi_ponto*dt;

% Encontra velocidade linear em relação ao body axis
vel_linear_body = vel_linear_body + a*dt;

XYZ_ponto_ponto = matrizRotacao*a;

% Encontra velocidade linear em relação ao eixo inercial
XYZ_ponto = matrizRotacao*vel_linear_body;

% Encontra posição em relação ao eixo inercial
XYZ = XYZ+XYZ_ponto*dt;

estados = horzcat(XYZ, XYZ_ponto, phi_theta_psi, phi_theta_psi_ponto);

== matlab function VTOL/Atuador/Motor mixer ==
  data: u1thrust input; w1 output; u2mRoll input; u3mPitch input; u4mYaw input; w2 output; w3 output; w4 output; ktd input; kdd input; lb input
% Transforma um comando de thrust e momento em velocidade angular
function [w1,w2,w3,w4]= fcn(u1thrust, u2mRoll, u3mPitch, u4mYaw, ktd, kdd, lb)
% Supondo que U seja força e momentos
%w2ParaU = [ Ktd      Ktd     Ktd      Ktd;
%          -Ktd*Lb   Ktd*Lb  Ktd*Lb  -Ktd*Lb;
%           Ktd*Lb  -Ktd*Lb  Ktd*Lb  -Ktd*Lb;
%          -Kdd     -Kdd     Kdd      Kdd]

w2ParaU = [ ktd      ktd     ktd      ktd;
           -ktd*lb(2)      ktd*lb(1)     ktd*lb(1)     -ktd*lb(2);
            ktd*lb(3)     -ktd*lb(4)     ktd*lb(3)     -ktd*lb(4);
           -kdd     -kdd       kdd      kdd];


w = inv(w2ParaU)*[u1thrust ; u2mRoll ; u3mPitch ; u4mYaw];
for i = 1:numel(w);
   if(w(i) > 837.75^2)
      w(i) = 837.75^2; 
   end
end
for i = 1:numel(w);
   if(w(i) < 0)
      w(i) = 0; 
   end
end

w1 = sqrt(w(1));
w2 = sqrt(w(2));
w3 = sqrt(w(3));
w4 = sqrt(w(4));

== matlab function VTOL/Interface gráfica1/Desenho do drone ==
  data: desenhoDrone output
function desenhoDrone = fcn

%Retângulo com o espaçamento dos motores
%Braço Motor 1
p1 = [-0.54 -0.54 0];
p2 = [0.54 -0.54 0];
%Braço Motor 2
p3 = [0.54 0.54 0];
p4 = [-0.54 0.54 0]; 
%Braço quad
p5 = [0 -1 0];
p6 = [0 1 0];

%boom
p7 = [0 0 0];
p8 = [-1 0 0];

%profundor
p9 = [-1 -0.3 0];
p10 = [-1 0.3 0];

%leme
p11 = [-1 0 0];
p12 = [-1 0 0.3];

desenhoDrone = [[p1(1) p2(1) p3(1) p4(1) p5(1) p6(1) p7(1) p8(1) p9(1) p10(1) p11(1) p12(1)]; [p1(2) p2(2) p3(2) p4(2) p5(2) p6(2) p7(2) p8(2) p9(2) p10(2) p11(2) p12(2)]; [p1(3) p2(3) p3(3) p4(3) p5(3) p6(3) p7(3) p8(3) p9(3) p10(3) p11(3) p12(3)]];

== matlab function VTOL/Interface gráfica1/Rotacao ==
  data: vetorNoEixoDoCorpo input; vetorNoEixoInercial output; PitchRollYaw input; XYZ input
function vetorNoEixoInercial = fcn(vetorNoEixoDoCorpo, PitchRollYaw, XYZ)
pitch = PitchRollYaw(1);
roll = PitchRollYaw(2);
yaw = PitchRollYaw(3);


matrizRotacao =     [cos(pitch)*cos(yaw) sin(roll)*sin(pitch)*cos(yaw)-cos(roll)*sin(yaw) cos(roll)*sin(pitch)*cos(yaw)+sin(roll)*sin(yaw);
   cos(pitch)*sin(yaw) sin(roll)*sin(pitch)*sin(yaw)+cos(roll)*cos(yaw) cos(roll)*sin(pitch)*sin(yaw)-sin(roll)*cos(yaw);
   -sin(pitch) sin(roll)*cos(pitch) cos(roll)*cos(pitch)];

% matrizRotacao =     [cos(pitch)*cos(yaw) sin(roll)*sin(pitch)*cos(yaw)-cos(roll)*sin(yaw) cos(roll)*sin(pitch)*cos(yaw)+sin(roll)*sin(yaw);
%     cos(pitch)*sin(yaw) sin(roll)*sin(pitch)*sin(yaw)+cos(roll)*cos(yaw) cos(roll)*sin(pitch)*sin(yaw)-sin(roll)*cos(yaw);
%     -sin(pitch) sin(roll)*cos(pitch) cos(roll)*cos(pitch)]

vetorNoEixoInercial = matrizRotacao*vetorNoEixoDoCorpo;
vetorNoEixoInercial = vetorNoEixoInercial + repmat(XYZ,1,size(vetorNoEixoInercial, 2));

== matlab function VTOL/Interface gráfica1/desenhaVetores ==
  data: vetorNoEixoDoCorpo input; vetorNoEixoInercial input
function fcn(vetorNoEixoDoCorpo, vetorNoEixoInercial)
coder.extrinsic('quiver3');

coder.extrinsic('fill3');
%Desenha eixo Inercial
quiver3(0,0,0, 1, 0, 0);
hold on
quiver3(0,0,0, 0, 1, 0);
quiver3(0,0,0, 0, 0, 1);
vetorNoEixoInercial(1, :);

plot3(vetorNoEixoInercial(1, 1:2), vetorNoEixoInercial(2, 1:2), vetorNoEixoInercial(3, 1:2), 'LineWidth', 2, 'LineJoin', 'round');
plot3(vetorNoEixoInercial(1, 3:4), vetorNoEixoInercial(2, 3:4), vetorNoEixoInercial(3, 3:4), 'LineWidth', 2, 'LineJoin', 'round');
plot3(vetorNoEixoInercial(1, 5:6), vetorNoEixoInercial(2, 5:6), vetorNoEixoInercial(3, 5:6), 'LineWidth', 6, 'LineJoin', 'round');
plot3(vetorNoEixoInercial(1, 7:8), vetorNoEixoInercial(2, 7:8), vetorNoEixoInercial(3, 7:8), 'LineWidth', 3, 'LineJoin', 'round');
plot3(vetorNoEixoInercial(1, 9:10), vetorNoEixoInercial(2, 9:10), vetorNoEixoInercial(3, 9:10), 'LineWidth', 3, 'LineJoin', 'round');
plot3(vetorNoEixoInercial(1, 11:12), vetorNoEixoInercial(2, 11:12), vetorNoEixoInercial(3, 11:12), 'LineWidth', 3, 'LineJoin', 'round');
xlabel('x'); ylabel('y'); zlabel('z');  

axis([-10 10 -10 10 -1 10]);
hold off
